simulink model "Diesel_UnitTest"  (Simulink 8.7)
settings: Solver=ode1  StartTime=0.0  StopTime=inf  FixedStep=Ts  MaxStep=1e-3  RelTol=1e-3
model workspace (MAT data in the model file):
  op_snapshot1 : opcond.OperatingPoint (value not decoded)
PostLoadFcn:
  | Test_init;
InitFcn:
  | Test_init;
values from neighbouring files (symbols this model uses):
  Ts = 100E-6    (= 0.0001)    [Test_init.m]
undefined symbols (not defined in the file or in its folder): Banshee_HWCtrl_IOs, Banshee_SEL751_Woodward_lib, fdesignblkfcn, gcbh, Left, type, V
libraries: simulink x11, rtio_opalrt_common x10, cables_lib x7, rtlab x6, breaker_lib x5, simulink_extras x3, Load_lib x3, PQFV_lib x2, powerlib x2, artemis x1, EasyGen3500_GensetSignalScaling_lib x1, HWController_Diesel_GenSet_4MVA_lib x1
(part 1 of 2)
settings Model: ARTEMISmethode_block_infos=$$__separator__$$Diesel_UnitTest/ARTEMIS Guide$$__separator__$$  Creator=RE25624  LastModifiedBy=g73labuser
settings SolverCC: ZeroCrossAlgorithm=Adaptive
settings DataIOCC: ExternalInput=getinputstruct(op_snapshot1)  InitialState=getstatestruct(op_snapshot1)  LimitDataPoints=off  MaxDataPoints=90060  SaveOutput=off  SignalLogging=off  DSMLogging=off  SaveTime=off  OutputSaveName=result
settings OptimizationCC: BlockReduction=off  OptimizeBlockIOStorage=off  BufferReuse=off  GlobalBufferReuse=off  ExpressionFolding=off  ExpressionDepthLimit=2147483647  LocalBlockOutputs=off
settings DebuggingCC: MaxConsecutiveZCsMsg=warning  IgnoredZcDiagnostic=none  MultiTaskRateTransMsg=warning  FcnCallInpInsideContextMsg=EnableAllAsWarning  ModelReferenceExtraNoncontSigs=warning  StateNameClashWarn=warning  StrictBusMsg=None
settings ModelReferenceCC: UpdateModelReferenceTargets=IfOutOfDate
settings SFSimCC: SFSimEcho=off
settings GRTTargetCC: CombineOutputUpdateFcns=off  GRTInterface=on

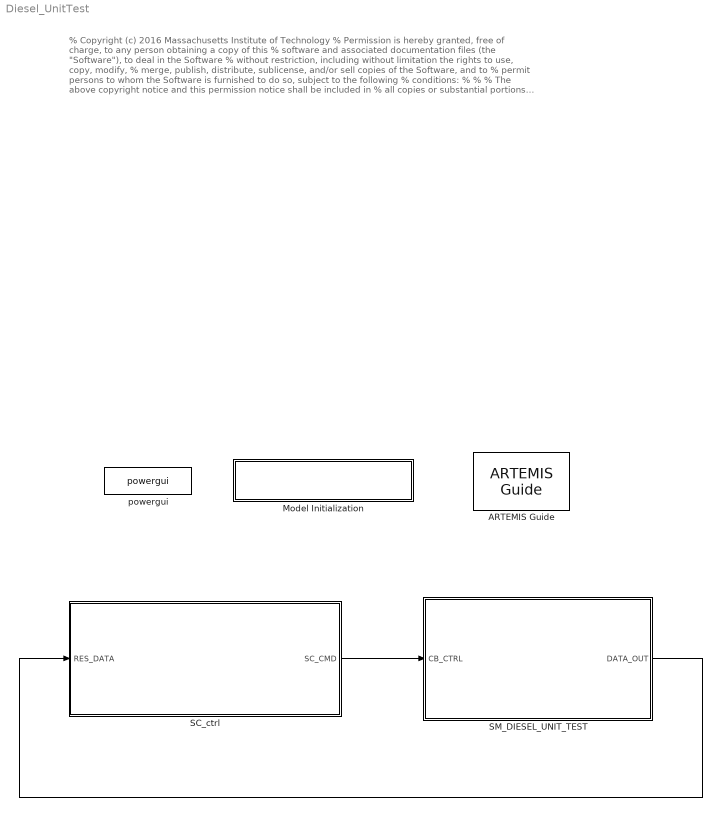
== system Diesel_UnitTest ==
  note: % Copyright (c) 2016 Massachusetts Institute of Technology
      | % Permission is hereby granted, free of charge, to any person obtaining a copy of this
      | % software and associated documentation files (the "Software"), to deal in the Software
      | % without restriction, including without limitation the rights to use, copy, modify,
      | % merge, publish, distribute, sublicense, and/or sell copies of the Software, and to
      | % permit persons to whom the Software is furnished to do so, subject to the following
      | % conditions:
      | %
      | %
      | % The above copyright notice and this permission notice shall be included in
      | % all copies or substantial portions of the Software.
      | %
      | % THE SOFTWARE IS PROVIDED "AS IS", WITHOUT WARRANTY OF ANY KIND, EXPRESS OR IMPLIED,
      | % INCLUDING BUT NOT LIMITED TO THE WARRANTIES OF MERCHANTABILITY, FITNESS FOR A
      | % PARTICULAR PURPOSE AND NONINFRINGEMENT. IN NO EVENT SHALL THE AUTHORS OR COPYRIGHT
      | % HOLDERS BE LIABLE FOR ANY CLAIM, DAMAGES OR OTHER LIABILITY, WHETHER IN AN ACTION
      | % OF CONTRACT, TORT OR OTHERWISE, ARISING FROM, OUT OF OR IN CONNECTION WITH THE
      | % SOFTWARE OR THE USE OR OTHER DEALINGS IN THE SOFTWARE.
      | %
      | %
      | %%
  ARTEMIS Guide : artemis/ARTEMIS/ARTEMIS Guide  Tag=FTSSmethode_opal_4hx0r99  Description=5.0_z1  lock=on  Ts=Ts  opt=art5  dyna=off  nb_perm=4  RT_fullcomp=off  ssn=on  ssn_itvc=off  ssn_ivic=off  ssn_ext=off  ssn_solver=Art5 with Backward Euler nodal interface  ssn_impulse=off  ssn_quasimpulse=off  ssn_impulse_loop=5  paraExtinctionThy=off  Thy_Impulse=on  dtc=Off  dtc_opt=normal  ao=on  simtype=off  ct_mac=off  lin_mov=off  lsp=[0.001 2]  spike_skip=Disabled  dtc_extra=1  dtc_sws=normal  dtc_pied=0.5  SPSRulesBlock=SPSRules  tre=on  ctmm=off  LF=off  dpl_type=ARTEMiS DPL  rlc_type=off  custom_type=off  para=on  ssn_ImpulseLoopBlockedStateUpdate=5  ssn_mov_iter_number=5  ssn_switch_iter_number=5  ssn_nib_type_verify=on  ssn_use_lu=on  ssn_use_ldlt=off
  Model Initialization : Subsystem  AncestorBlock=artemis/Tools /Misc/Model Initialization  mask(Model Functions){InitFcnX=Test_init;, prel=off, posl=on, inif=on, strf=off}
      mask prompts: InitFcnX "Initialisation"; prel "Preload Function"; posl "PostLoad Function"; inif "InitFcn"; strf "StartFcn"
      mask init:
      | currentBlock = gcb;
      | root = bdroot(currentBlock);
      | 
      | if ~strcmp(get_param(root,'BlockDiagramType'),'library')
      |     if prel==1
      |         set_param(root, 'PreLoadFcn', InitFcnX);
      |     else
      |         set_param(root, 'PreLoadFcn', '');
      |     end
      |     if inif==1
      |         set_param(root, 'InitFcn', InitFcnX);
      |     else
      |         set_param(root, 'InitFcn', '');
      |     end
      |     if strf==1
      |         set_param(root, 'StartFcn', InitFcnX);
      |     else
      |         set_param(root, 'StartFcn', '');
      |     end
      |     if posl==1
      |         set_param(root, 'PostLoadFcn', InitFcnX);
      |     else
      |         set_param(root, 'PostLoadFcn', '');
      |     end
      | end
      | 
      | pos = get_param(currentBlock, 'Position');
      | width = pos(3) - pos(1); height = pos(4) - pos(2);
      | txt = [ upper(root) '\n' '- InitFcn. . . . . '  get_param(root, 'InitFcn') ];
      settings: CopyFcn=set_param(gcb,'LinkStatus','inactive')
      mask Display: text(5, height*0.5, txt, 'horizontalAlignment', 'left', 'verticalAlignment', 'middle') ;
  SC_ctrl : Subsystem
  SM_DIESEL_UNIT_TEST : Subsystem
  powergui : powerlib/powergui  Priority=2  SimulationMode=Discrete  SolverType=Tustin  SampleTime=Ts  frequency=60  SPID=off  DisableSnubberDevices=off  DisableRonSwitches=off  DisableVfSwitches=off  SwTol=0  DisplayEquations=off  Interpol=off  ExternalGateDelay=off  methode=off  Ts=0  FunctionMessages=off  echomessages=off  HookPort=off  EnableUseOfTLC=off  x0status=blocks  frequencyindice=0  Pbase=100e6  ErrMax=1e-4  Iterations=50  UnitsV=kV  UnitsW=MW  buscounter=0  RestoreLinks=warning  ResistiveCurrentMeasurement=off  Frange=logspace(0,3,50)  Ylog=off  Xlog=off  ShowGrid=off  save=off  variable=ZData  structure=0  ZoomFFT=on  StartTime=0.0  cycles=2  DisplayStyle=off  fundamental=60  FreqAxis=off  MaxFrequency=1000  frequencyindicesteady=1  RmsSteady=1  display=off
  wires:
  SC_ctrl/1(SC_CMD) -> SM_DIESEL_UNIT_TEST/1(CB_CTRL)
  SM_DIESEL_UNIT_TEST/1(DATA_OUT) -> SC_ctrl/1(RES_DATA)

== system Diesel_UnitTest/Model Initialization ==

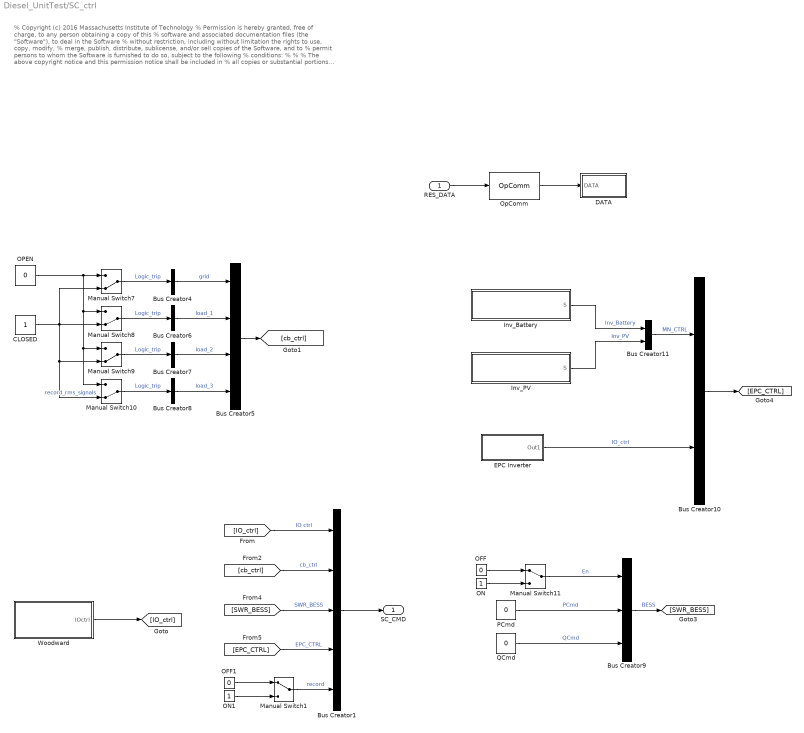
== system Diesel_UnitTest/SC_ctrl ==
  note: % Copyright (c) 2016 Massachusetts Institute of Technology
      | % Permission is hereby granted, free of charge, to any person obtaining a copy of this
      | % software and associated documentation files (the "Software"), to deal in the Software
      | % without restriction, including without limitation the rights to use, copy, modify,
      | % merge, publish, distribute, sublicense, and/or sell copies of the Software, and to
      | % permit persons to whom the Software is furnished to do so, subject to the following
      | % conditions:
      | %
      | %
      | % The above copyright notice and this permission notice shall be included in
      | % all copies or substantial portions of the Software.
      | %
      | % THE SOFTWARE IS PROVIDED "AS IS", WITHOUT WARRANTY OF ANY KIND, EXPRESS OR IMPLIED,
      | % INCLUDING BUT NOT LIMITED TO THE WARRANTIES OF MERCHANTABILITY, FITNESS FOR A
      | % PARTICULAR PURPOSE AND NONINFRINGEMENT. IN NO EVENT SHALL THE AUTHORS OR COPYRIGHT
      | % HOLDERS BE LIABLE FOR ANY CLAIM, DAMAGES OR OTHER LIABILITY, WHETHER IN AN ACTION
      | % OF CONTRACT, TORT OR OTHERWISE, ARISING FROM, OUT OF OR IN CONNECTION WITH THE
      | % SOFTWARE OR THE USE OR OTHER DEALINGS IN THE SOFTWARE.
      | %
      | %
      | %%
  RES_DATA : Inport
  Bus Creator1 : BusCreator  Inputs=5
  Bus Creator10 : BusCreator  Inputs=2
  Bus Creator11 : BusCreator  Inputs=2
  Bus Creator{4,6..8} (4 alike) : BusCreator  Inputs=1
  Bus Creator5 : BusCreator  Inputs=4
  Bus Creator9 : BusCreator  Inputs=3
  CLOSED : Constant
  DATA : Subsystem
  EPC Inverter : Subsystem
  Inv_Battery : Subsystem
  Inv_PV : Subsystem
  Manual Switch1 : ManualSwitch
  Manual Switch{7..10} (4 alike) : ManualSwitch  CurrentSetting=0
  Manual Switch11 : ManualSwitch
  OFF : Constant  Value=0
  OFF1 : Constant  Value=0
  ON : Constant
  ON1 : Constant
  OPEN : Constant  Value=0
  OpComm : rtlab/OpComm  nbport=1  groupe_acq=1  subsys_rate=0  st=0  Synchronization=on  Interpolation=on  Threshold=1.0  Missed_Data=off  Sim_Time=off  Samples=off  dynSigOut=off  from_console=0  warning_done=off  writeOpCommFile=off  Offset=off
  PCmd : Constant  Value=0  SampleTime=Ts
  QCmd : Constant  Value=0  SampleTime=Ts
  Woodward : Subsystem
  SC_CMD : Outport
  wires:
  Bus Creator1/1 -> SC_CMD/1
  [IO_ctrl] -> Bus Creator1/1  "IO ctrl"
  Woodward/1(IOctrl) -> [IO_ctrl]
  [cb_ctrl] -> Bus Creator1/2  "cb_ctrl"
  OpComm/1 -> DATA/1(DATA)
  RES_DATA/1 -> OpComm/1
  Manual Switch10/1 -> Bus Creator8/1  "Logic_trip"
  Manual Switch9/1 -> Bus Creator7/1  "Logic_trip"
  Bus Creator5/1 -> [cb_ctrl]
  Manual Switch8/1 -> Bus Creator6/1  "Logic_trip"
  Bus Creator4/1 -> Bus Creator5/1  "grid"
  Manual Switch7/1 -> Bus Creator4/1  "Logic_trip"
  Bus Creator8/1 -> Bus Creator5/4  "load_3"
  Bus Creator7/1 -> Bus Creator5/3  "load_2"
  Bus Creator6/1 -> Bus Creator5/2  "load_1"
  OPEN/1 -> Manual Switch7/1, Manual Switch8/1, Manual Switch9/1, Manual Switch10/1
  CLOSED/1 -> Manual Switch7/2, Manual Switch8/2, Manual Switch9/2, Manual Switch10/2  "record_rms_signals"
  Manual Switch11/1 -> Bus Creator9/1  "En"
  PCmd/1 -> Bus Creator9/2  "PCmd"
  QCmd/1 -> Bus Creator9/3  "QCmd"
  ON/1 -> Manual Switch11/2
  OFF/1 -> Manual Switch11/1
  Bus Creator9/1 -> [SWR_BESS]  "BESS"
  [SWR_BESS] -> Bus Creator1/3  "SWR_BESS"
  EPC Inverter/1(Out1) -> Bus Creator10/2  "IO_ctrl"
  Bus Creator10/1 -> [EPC_CTRL]
  [EPC_CTRL] -> Bus Creator1/4  "EPC_CTRL"
  Inv_Battery/1(S) -> Bus Creator11/1  "Inv_Battery"
  Bus Creator11/1 -> Bus Creator10/1  "MN_CTRL"
  Inv_PV/1(S) -> Bus Creator11/2  "Inv_PV"
  ON1/1 -> Manual Switch1/2
  OFF1/1 -> Manual Switch1/1
  Manual Switch1/1 -> Bus Creator1/5  "record"

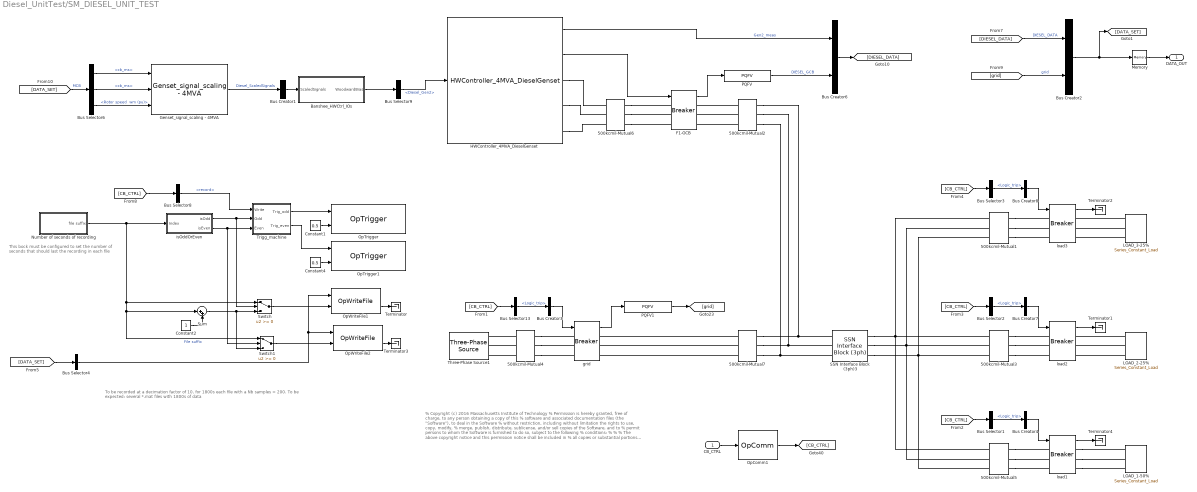
== system Diesel_UnitTest/SM_DIESEL_UNIT_TEST ==
  note: % Copyright (c) 2016 Massachusetts Institute of Technology
      | % Permission is hereby granted, free of charge, to any person obtaining a copy of this
      | % software and associated documentation files (the "Software"), to deal in the Software
      | % without restriction, including without limitation the rights to use, copy, modify,
      | % merge, publish, distribute, sublicense, and/or sell copies of the Software, and to
      | % permit persons to whom the Software is furnished to do so, subject to the following
      | % conditions:
      | %
      | %
      | % The above copyright notice and this permission notice shall be included in
      | % all copies or substantial portions of the Software.
      | %
      | % THE SOFTWARE IS PROVIDED "AS IS", WITHOUT WARRANTY OF ANY KIND, EXPRESS OR IMPLIED,
      | % INCLUDING BUT NOT LIMITED TO THE WARRANTIES OF MERCHANTABILITY, FITNESS FOR A
      | % PARTICULAR PURPOSE AND NONINFRINGEMENT. IN NO EVENT SHALL THE AUTHORS OR COPYRIGHT
      | % HOLDERS BE LIABLE FOR ANY CLAIM, DAMAGES OR OTHER LIABILITY, WHETHER IN AN ACTION
      | % OF CONTRACT, TORT OR OTHERWISE, ARISING FROM, OUT OF OR IN CONNECTION WITH THE
      | % SOFTWARE OR THE USE OR OTHER DEALINGS IN THE SOFTWARE.
      | %
      | %
      | %%
  note: This bock must be configured to set the number of
      | seconds that should last the recording in each file
  note: To be recorded at a decimation factor of 10,   for 1800s each file with a Nb samples = 200.
      | To be expected: several *.mat files with 1800s of data
  CB_CTRL : Inport
  500kcmil-Mutual1 : cables_lib/500kcmil-Mutual  length=500  par_sets=1  ratio=3
  500kcmil-Mutual{2,4,6..7} (4 alike) : cables_lib/500kcmil-Mutual  length=50  par_sets=1  ratio=3
  500kcmil-Mutual3 : cables_lib/500kcmil-Mutual  length=500  par_sets=1  ratio=3
  500kcmil-Mutual5 : cables_lib/500kcmil-Mutual  length=500  par_sets=1  ratio=3
  Banshee_HWCtrl_IOs : Subsystem  AncestorBlock=Banshee_SEL751_Woodward_lib/Banshee_HWCtrl_IOs
  Bus Creator{1,3..4,7..8} (5 alike) : BusCreator  Inputs=1
  Bus Creator2 : BusCreator  Inputs=2
  Bus Creator6 : BusCreator  Inputs=2
  Bus Selector1 : BusSelector  OutputSignals=cb_ctrl.load_1.Logic_trip
  Bus Selector13 : BusSelector  OutputSignals=cb_ctrl.grid.Logic_trip
  Bus Selector2 : BusSelector  OutputSignals=cb_ctrl.load_2.Logic_trip
  Bus Selector3 : BusSelector  OutputSignals=cb_ctrl.load_3.Logic_trip
  Bus Selector4 : BusSelector  OutputSignals="DIESEL_DATA.Gen2_meas.w.w.Rotor speed  wm (pu),DIESEL_DATA.Gen2_meas.Pm,DIESEL_DATA.DIESEL_GCB.VRMSLL,DIESEL_DATA.DIESEL_GCB.Freq,DIESEL_DATA.DIESEL_GCB.kw,DIESEL_DATA.DIESEL_GCB.kvar,DIESEL_DATA.DIESEL_GCB.cb_ms.Status,grid.VRMSLL,grid.Freq,grid.kw,grid.kvar,grid.cb_ms.Status"  OutputAsBus=on
  Bus Selector6 : BusSelector  OutputSignals="DIESEL_DATA.DIESEL_GCB.cb_ms,grid.cb_ms,DIESEL_DATA.Gen2_meas.w.w.Rotor speed  wm (pu)"
  Bus Selector8 : BusSelector  OutputSignals=record
  Bus Selector9 : BusSelector  OutputSignals=Diesel_Gen2
  Constant1 : Constant  Value=0.5
  Constant2 : Constant
  Constant4 : Constant  Value=0.5
  F1-GCB : breaker_lib/Breaker  Ts=Ts  mech_delay=cb_mech_delay
  Genset_signal_scaling - 4MVA : EasyGen3500_GensetSignalScaling_lib/Genset_signal_scaling - 4MVA  Vpk_mcb=11268  watt_mcb=3600000  Vpk_gcb=11268  watt_gcb=3600000  rated_rpm=1800  wm_noise_bias=0.02
  HWController_4MVA_DieselGenset : HWController_Diesel_GenSet_4MVA_lib/HWController_4MVA_DieselGenset
  LOAD_1-50% : Load_lib/Series_Constant_Load  v=13800  kVA=2000  pf=0.90
  LOAD_2-25% : Load_lib/Series_Constant_Load  v=13800  kVA=1000  pf=0.90
  LOAD_3-25% : Load_lib/Series_Constant_Load  v=13800  kVA=1000  pf=0.90
  Memory : Memory
  Number of seconds of recording : Subsystem  mask{time_s=1800}
      mask prompts: time_s "Time in seconds"
      mask help: Set the number of seconds that should last the recording in each file.
  OpComm1 : rtlab/OpComm  nbport=1  groupe_acq=1  subsys_rate=0  st=0  Synchronization=on  Interpolation=on  Threshold=1.0  Missed_Data=off  Sim_Time=off  Samples=off  dynSigOut=off  from_console=1  warning_done=off  writeOpCommFile=off  Offset=off
  OpTrigger : rtlab/DataLogging/OpTrigger  Trig_Type=TRIGGER SIGNAL >= TRIGGER LEVEL  Trig_Offset=0  Acq_Group=28
  OpTrigger1 : rtlab/DataLogging/OpTrigger  Trig_Type=TRIGGER SIGNAL >= TRIGGER LEVEL  Trig_Offset=0  Acq_Group=29
  OpWriteFile1 : rtlab/DataLogging/OpWriteFile  Static_File=off  varname=recVar  Filename=A_FILE_RECORDED_o.mat  rtpath='./'  nrtpath='.\'  Acq_Group=28  file_size=150000000  write_offline=off  Sim_Mode=off  Nb_Samples=1000  Buffer_size=0
      settings: Decimation=20
  OpWriteFile2 : rtlab/DataLogging/OpWriteFile  Static_File=off  varname=recVar  Filename=A_FILE_RECORDED_e.mat  rtpath='./'  nrtpath='.\'  Acq_Group=29  file_size=150000000  write_offline=off  Sim_Mode=off  Nb_Samples=1000  Buffer_size=0
      settings: Decimation=20
  PQFV : PQFV_lib/PQFV  VRMSLL=13800  Ts=Ts
  PQFV1 : PQFV_lib/PQFV  VRMSLL=13800  Ts=Ts
  SSN Interface Block (3ph)3 : ssn_lib/SSN Interface Block (3ph)  nb_phase=3  nb_port=2  p1_type=V-type(Left)  p2_type=V-type (Right)  p3_type=V-type(Left)  p4_type=V-type(Left)  p5_type=V-type(Left)  p6_type=V-type(Left)  p7_type=V-type(Left)  p8_type=V-type(Left)  p9_type=V-type(Left)  p10_type=V-type(Left)  p11_type=V-type(Left)  p12_type=V-type(Left)  p13_type=V-type(Left)  p14_type=V-type(Left)  p15_type=V-type(Left)  p16_type=V-type(Left)  I_port_shunt_resistance=1e9
  Sum : Sum  Inputs=|++
  Switch : Switch
  Switch1 : Switch
  Terminator{,1..4} (5 alike) : Terminator
  Three-Phase Source1 : powerlib/Electrical Sources/Three-Phase Source  InternalConnection=Yg  VoltagePhases=off  Voltage=13800 * 1.02  PhaseAngle=0  Voltage_phases=[25e3 25e3 25e3]/sqrt(3)  PhaseAngles_phases=[0 -120 +120]  Frequency=60  NonIdealSource=on  SpecifyImpedance=on  Resistance=0.8929  Inductance=16.58e-3  ShortCircuitLevel=2000e6  BaseVoltage=13800 * 1.02  XRratio=100  BusType=swing  Pref=0  Qref=0  Prefabc=[10e3, 10e3, 10e3]  Qrefabc=[0, 0, 0]  Qmin=-inf  Qmax=inf
  Trigg_machine : Subsystem
  grid : breaker_lib/Breaker  Ts=Ts  mech_delay=cb_mech_delay
  isOddOrEven : Subsystem
  load1 : breaker_lib/Breaker  Ts=Ts  mech_delay=cb_mech_delay
  load2 : breaker_lib/Breaker  Ts=Ts  mech_delay=cb_mech_delay
  load3 : breaker_lib/Breaker  Ts=Ts  mech_delay=cb_mech_delay
  DATA_OUT : Outport
  wires:
  Bus Selector9/1 -> HWController_4MVA_DieselGenset/1  "<Diesel_Gen2>"
  HWController_4MVA_DieselGenset/2 -> F1-GCB/1
  F1-GCB/1 -> PQFV/1
  Bus Creator6/1 -> [DIESEL_DATA]
  PQFV/1 -> Bus Creator6/2  "DIESEL_GCB"
  HWController_4MVA_DieselGenset/1 -> Bus Creator6/1  "Gen2_meas"
  Memory/1 -> DATA_OUT/1
  Bus Creator2/1 -> [DATA_SET], Memory/1
  [DIESEL_DATA] -> Bus Creator2/1  "DIESEL_DATA"
  [grid] -> Bus Creator2/2  "grid"
  [CB_CTRL] -> Bus Selector13/1
  Bus Selector13/1 -> Bus Creator3/1  "<Logic_trip>"
  Bus Creator3/1 -> grid/1
  grid/1 -> PQFV1/1
  PQFV1/1 -> [grid]
  [CB_CTRL] -> Bus Selector1/1
  Bus Selector1/1 -> Bus Creator4/1  "<Logic_trip>"
  Bus Creator4/1 -> load1/1
  [CB_CTRL] -> Bus Selector2/1
  Bus Selector2/1 -> Bus Creator7/1  "<Logic_trip>"
  Bus Creator7/1 -> load2/1
  [CB_CTRL] -> Bus Selector3/1
  Bus Selector3/1 -> Bus Creator8/1  "<Logic_trip>"
  Bus Creator8/1 -> load3/1
  load1/1 -> Terminator4/1
  load3/1 -> Terminator2/1
  load2/1 -> Terminator1/1
  Bus Selector4/1 -> OpWriteFile1/1, OpWriteFile2/1
  Trigg_machine/1(Trig_odd) -> OpTrigger/1
  Trigg_machine/2(Trig_even) -> OpTrigger1/1
  Constant1/1 -> OpTrigger/2
  Constant4/1 -> OpTrigger1/2
  isOddOrEven/1(isOdd) -> Switch/2, Trigg_machine/2(Odd)
  isOddOrEven/2(isEven) -> Switch1/2, Trigg_machine/3(Even)
  Switch/1 -> OpWriteFile1/2
  Switch1/1 -> OpWriteFile2/2
  Constant2/1 -> Sum/2
  Sum/1 -> Switch/3, Switch1/3
  Number of seconds of recording/1(file suffix) -> isOddOrEven/1(Index), Sum/1, Switch1/1, Switch/1  "File suffix"
  Bus Selector8/1 -> Trigg_machine/1(Write)  "<record>"
  OpWriteFile1/2 -> Terminator/1
  OpWriteFile2/2 -> Terminator3/1
  [CB_CTRL] -> Bus Selector8/1
  [DATA_SET] -> Bus Selector4/1
  CB_CTRL/1 -> OpComm1/1
  OpComm1/1 -> [CB_CTRL]
  [DATA_SET] -> Bus Selector6/1  "MCB"
  Bus Selector6/3 -> Genset_signal_scaling - 4MVA/3  "<Rotor speed  wm (pu)>"
  Bus Selector6/2 -> Genset_signal_scaling - 4MVA/2  "<cb_ms>"
  Bus Selector6/1 -> Genset_signal_scaling - 4MVA/1  "<cb_ms>"
  Genset_signal_scaling - 4MVA/1 -> Bus Creator1/1  "Diesel_ScaledSignals"
  Bus Creator1/1 -> Banshee_HWCtrl_IOs/1(ScaledSignals)
  Banshee_HWCtrl_IOs/1(WoodwardBias) -> Bus Selector9/1
  connections:
  500kcmil-Mutual6/RConn3 -- F1-GCB/LConn3
  500kcmil-Mutual6/RConn1 -- F1-GCB/LConn1
  500kcmil-Mutual6/RConn2 -- F1-GCB/LConn2
  HWController_4MVA_DieselGenset/RConn1 -- 500kcmil-Mutual6/LConn1
  HWController_4MVA_DieselGenset/RConn2 -- 500kcmil-Mutual6/LConn2
  HWController_4MVA_DieselGenset/RConn3 -- 500kcmil-Mutual6/LConn3
  500kcmil-Mutual4/LConn2 -- Three-Phase Source1/RConn2
  500kcmil-Mutual4/LConn1 -- Three-Phase Source1/RConn1
  500kcmil-Mutual4/LConn3 -- Three-Phase Source1/RConn3
  load1/RConn2 -- LOAD_1-50%/LConn2
  load1/RConn3 -- LOAD_1-50%/LConn3
  load1/RConn1 -- LOAD_1-50%/LConn1
  LOAD_2-25%/LConn1 -- load2/RConn1
  LOAD_2-25%/LConn2 -- load2/RConn2
  LOAD_2-25%/LConn3 -- load2/RConn3
  LOAD_3-25%/LConn3 -- load3/RConn3
  LOAD_3-25%/LConn1 -- load3/RConn1
  LOAD_3-25%/LConn2 -- load3/RConn2
  500kcmil-Mutual1/RConn3 -- load3/LConn3
  500kcmil-Mutual1/RConn2 -- load3/LConn2
  500kcmil-Mutual1/RConn1 -- load3/LConn1
  500kcmil-Mutual3/RConn1 -- load2/LConn1
  500kcmil-Mutual3/RConn3 -- load2/LConn3
  500kcmil-Mutual3/RConn2 -- load2/LConn2
  500kcmil-Mutual5/RConn1 -- load1/LConn1
  500kcmil-Mutual5/RConn3 -- load1/LConn3
  500kcmil-Mutual5/RConn2 -- load1/LConn2
  500kcmil-Mutual2/LConn3 -- F1-GCB/RConn3
  500kcmil-Mutual2/LConn2 -- F1-GCB/RConn2
  500kcmil-Mutual2/LConn1 -- F1-GCB/RConn1
  500kcmil-Mutual4/RConn2 -- grid/LConn2
  500kcmil-Mutual4/RConn3 -- grid/LConn3
  500kcmil-Mutual4/RConn1 -- grid/LConn1
  500kcmil-Mutual7/LConn2 -- grid/RConn2
  500kcmil-Mutual7/LConn3 -- grid/RConn3
  500kcmil-Mutual7/LConn1 -- grid/RConn1
  500kcmil-Mutual7/RConn3 -- 500kcmil-Mutual2/RConn3 -- SSN Interface Block (3ph)3/LConn3
  500kcmil-Mutual7/RConn2 -- 500kcmil-Mutual2/RConn2 -- SSN Interface Block (3ph)3/LConn2
  500kcmil-Mutual7/RConn1 -- 500kcmil-Mutual2/RConn1 -- SSN Interface Block (3ph)3/LConn1
  SSN Interface Block (3ph)3/RConn1 -- 500kcmil-Mutual1/LConn1 -- 500kcmil-Mutual5/LConn1 -- 500kcmil-Mutual3/LConn1
  SSN Interface Block (3ph)3/RConn3 -- 500kcmil-Mutual5/LConn3 -- 500kcmil-Mutual1/LConn3 -- 500kcmil-Mutual3/LConn3
  SSN Interface Block (3ph)3/RConn2 -- 500kcmil-Mutual5/LConn2 -- 500kcmil-Mutual1/LConn2 -- 500kcmil-Mutual3/LConn2

== system Diesel_UnitTest/SC_ctrl/DATA ==
  DATA : Inport
  Bus Selector : BusSelector  OutputSignals="DIESEL_DATA.DIESEL_GCB.Freq,DIESEL_DATA.Gen2_meas.w.w.Rotor speed  wm (pu),DIESEL_DATA.DIESEL_GCB.Vpu,DIESEL_DATA.DIESEL_GCB.kw,grid.kw,DIESEL_DATA.DIESEL_GCB.kvar,grid.kvar"
  Demux{,1..3} (4 alike) : Demux  Outputs=1
  Display : Display
  Mux : Mux  Inputs=2
  Mux1 : Mux  Inputs=2
  Mux2 : Mux  Inputs=2
  Scope : Scope  NumInputPorts=4
  wires:
  DATA/1 -> Bus Selector/1
  Bus Selector/1 -> Scope/1, Display/1  "<Freq>"
  Bus Selector/3 -> Mux/2  "<Vpu>"
  Bus Selector/2 -> Mux/1  "<Rotor speed  wm (pu)>"
  Mux/1 -> Scope/2
  Bus Selector/4 -> Demux/1  "<kw>"
  Bus Selector/5 -> Demux1/1  "<kw>"
  Mux1/1 -> Scope/3
  Bus Selector/6 -> Demux2/1  "<kvar>"
  Bus Selector/7 -> Demux3/1  "<kvar>"
  Mux2/1 -> Scope/4
  Demux/1 -> Mux1/1  "genset_kW"
  Demux1/1 -> Mux1/2  "grid_kW"
  Demux2/1 -> Mux2/1  "genset_kVAR"
  Demux3/1 -> Mux2/2  "grid_kW"

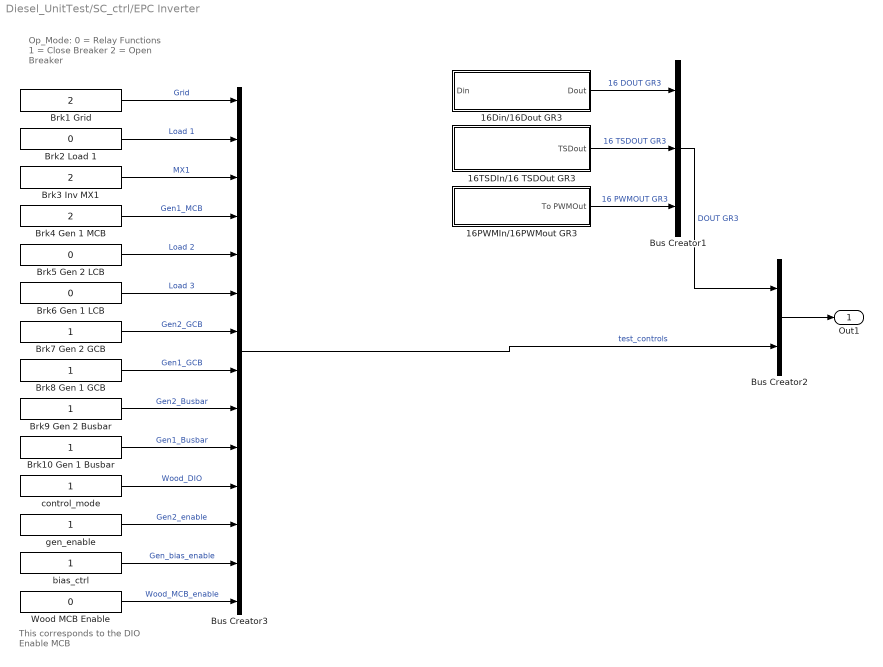
== system Diesel_UnitTest/SC_ctrl/EPC Inverter ==
  note: This corresponds to
      | the DIO Enable MCB
  note: Op_Mode:
      | 0 = Relay Functions
      | 1 = Close Breaker
      | 2 = Open Breaker
  16Din/16Dout GR3 : Subsystem
  16PWMIn/16PWMout GR3 : Subsystem
  16TSDIn/16 TSDOut GR3 : Subsystem
  Brk1 Grid : Constant  Value=2
  Brk10 Gen 1 Busbar : Constant
  Brk2 Load 1 : Constant  Value=0
  Brk3 Inv MX1 : Constant  Value=2
  Brk4 Gen 1 MCB : Constant  Value=2
  Brk5 Gen 2 LCB : Constant  Value=0
  Brk6 Gen 1 LCB : Constant  Value=0
  Brk7 Gen 2 GCB : Constant
  Brk8 Gen 1 GCB : Constant
  Brk9 Gen 2 Busbar : Constant
  Bus Creator1 : BusCreator  Inputs=3
  Bus Creator2 : BusCreator  Inputs=2
  Bus Creator3 : BusCreator  Inputs=14
  Wood MCB Enable : Constant  Value=0
  bias_ctrl : Constant
  control_mode : Constant
  gen_enable : Constant
  Out1 : Outport
  wires:
  Brk10 Gen 1 Busbar/1 -> Bus Creator3/10  "Gen1_Busbar"
  Brk9 Gen 2 Busbar/1 -> Bus Creator3/9  "Gen2_Busbar"
  Brk8 Gen 1 GCB/1 -> Bus Creator3/8  "Gen1_GCB"
  Brk7 Gen 2 GCB/1 -> Bus Creator3/7  "Gen2_GCB"
  Brk6 Gen 1 LCB/1 -> Bus Creator3/6  "Load 3"
  Brk5 Gen 2 LCB/1 -> Bus Creator3/5  "Load 2"
  Wood MCB Enable/1 -> Bus Creator3/14  "Wood_MCB_enable"
  Bus Creator2/1 -> Out1/1
  bias_ctrl/1 -> Bus Creator3/13  "Gen_bias_enable"
  gen_enable/1 -> Bus Creator3/12  "Gen2_enable"
  control_mode/1 -> Bus Creator3/11  "Wood_DIO"
  Brk4 Gen 1 MCB/1 -> Bus Creator3/4  "Gen1_MCB"
  Brk3 Inv MX1/1 -> Bus Creator3/3  "MX1"
  Brk2 Load 1/1 -> Bus Creator3/2  "Load 1"
  Brk1 Grid/1 -> Bus Creator3/1  "Grid"
  Bus Creator3/1 -> Bus Creator2/2  "test_controls"
  Bus Creator1/1 -> Bus Creator2/1  "DOUT GR3"
  16PWMIn/16PWMout GR3/1(To PWMOut) -> Bus Creator1/3  "16 PWMOUT GR3"
  16TSDIn/16 TSDOut GR3/1(TSDout) -> Bus Creator1/2  "16 TSDOUT GR3"
  16Din/16Dout GR3/1(Dout) -> Bus Creator1/1  "16 DOUT GR3"

== system Diesel_UnitTest/SC_ctrl/Inv_Battery ==
  note: Make this 1 to allow
      | the external signals.
  note: Remote Sense =>1
      | Use Remote Sense EPyQ
      | Sync or not => grid forming/grid following
  note: 0=> Local
      | 1=> Remote
  note: 0=> No Console
      | 1=> Console Ctrl
  note: 1 => Sig 1 is Bot then Sig 2 is Top
      | 0 => Sig 1 is Top then Sig 2 is Bot
  note: 0=> RTE
      | 1=> Simulink
  note: LSB
  note: MSB
  note: 1111: RTE TSD Signal Modulation External
      | 0111: RTE Signal Modulation Internal
      | X011: Sin Tri Modulatiion Internal
      | XX01: Digital Inputs
      | XXX0; Open Switches
  note: MCB
  note: GCB
  note: 1 => Closed
      | 0 => Open
  note: ~ 2.5 sec to get
      | to rated voltage
  note: RTE Internal
      | All 0 and one 1
  note: Internal = 0
      | External = 1
  Bus Creator : BusCreator  Inputs=8
  Bus Creator1 : BusCreator  Inputs=5
  Console : Constant  Value=0
  DC Contactor : Constant  Value=0
  Enable PWM{0..3} (4 alike) : Constant
  MX1 : Constant  Value=0
  MX2 : Constant  Value=0
  Precharge : Constant  Value=0
  Sense : Constant  Value=0
  Signal Mapping : Constant
  Simulink : Constant  Value=0
  S : Outport
  wires:
  Sense/1 -> Bus Creator/8  "LOCALvsREMOTE"
  Console/1 -> Bus Creator/7  "Console_Ctrl"
  Signal Mapping/1 -> Bus Creator1/5  "Ext_PWM_RTE_Signal"
  Simulink/1 -> Bus Creator/6  "RTEvsSPS"
  Enable PWM3/1 -> Bus Creator1/1
  Enable PWM2/1 -> Bus Creator1/2
  Enable PWM1/1 -> Bus Creator1/3
  Enable PWM0/1 -> Bus Creator1/4
  Bus Creator1/1 -> Bus Creator/1  "Enable PWM"
  MX2/1 -> Bus Creator/5  "MX2"
  MX1/1 -> Bus Creator/4  "MX1"
  DC Contactor/1 -> Bus Creator/3  "DC_Contactor"
  Precharge/1 -> Bus Creator/2  "Precharge"
  Bus Creator/1 -> S/1

== system Diesel_UnitTest/SC_ctrl/Inv_PV ==
  note: Make this 1 to allow
      | the external signals.
  note: Remote Sense =>1
      | Use Remote Sense EPyQ
      | Sync or not => grid forming/grid following
  note: 0=> Local
      | 1=> Remote
  note: 0=> No Console
      | 1=> Console Ctrl
  note: 1 => Sig 1 is Bot then Sig 2 is Top
      | 0 => Sig 1 is Top then Sig 2 is Bot
  note: 0=> RTE
      | 1=> Simulink
  note: LSB
  note: MSB
  note: 1111: RTE TSD Signal Modulation External
      | 0111: RTE Signal Modulation Internal
      | X011: Sin Tri Modulatiion Internal
      | XX01: Digital Inputs
      | XXX0; Open Switches
  note: MCB
  note: GCB
  note: 1 => Closed
      | 0 => Open
  note: ~ 2.5 sec to get
      | to rated voltage
  note: RTE Internal
      | All 0 and one 1
  note: Internal = 0
      | External = 1
  Bus Creator : BusCreator  Inputs=8
  Bus Creator1 : BusCreator  Inputs=5
  Console : Constant  Value=0
  DC Contactor : Constant  Value=0
  Enable PWM{0..3} (4 alike) : Constant
  MX1 : Constant  Value=0
  MX2 : Constant  Value=0
  Precharge : Constant  Value=0
  Sense : Constant  Value=0
  Signal Mapping : Constant
  Simulink : Constant  Value=0
  S : Outport
  wires:
  Sense/1 -> Bus Creator/8  "LOCALvsREMOTE"
  Console/1 -> Bus Creator/7  "Console_Ctrl"
  Signal Mapping/1 -> Bus Creator1/5  "Ext_PWM_RTE_Signal"
  Simulink/1 -> Bus Creator/6  "RTEvsSPS"
  Enable PWM3/1 -> Bus Creator1/1
  Enable PWM2/1 -> Bus Creator1/2
  Enable PWM1/1 -> Bus Creator1/3
  Enable PWM0/1 -> Bus Creator1/4
  Bus Creator1/1 -> Bus Creator/1  "Enable PWM"
  MX2/1 -> Bus Creator/5  "MX2"
  MX1/1 -> Bus Creator/4  "MX1"
  DC Contactor/1 -> Bus Creator/3  "DC_Contactor"
  Precharge/1 -> Bus Creator/2  "Precharge"
  Bus Creator/1 -> S/1

== system Diesel_UnitTest/SC_ctrl/Woodward ==
  16Din/16Dout GR3 : Subsystem
  Bus Creator2 : BusCreator  Inputs=1
  IOctrl : Outport
  wires:
  16Din/16Dout GR3/1(Dout) -> Bus Creator2/1  "16 DOUT GR3"
  Bus Creator2/1 -> IOctrl/1  "IO ctrl"

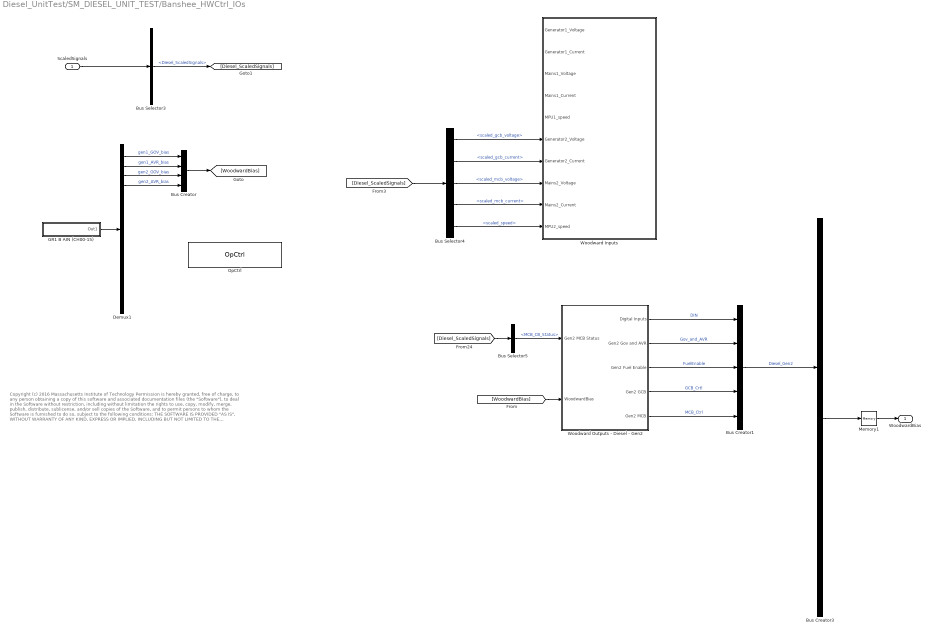
== system Diesel_UnitTest/SM_DIESEL_UNIT_TEST/Banshee_HWCtrl_IOs ==
  note: Copyright (c) 2016 Massachusetts Institute of Technology
      | Permission is hereby granted, free of charge, to any person obtaining a copy of this software and associated documentation files (the "Software"), to deal
      | in the Software without restriction, including without limitation the rights to use, copy, modify, merge, publish, distribute, sublicense, and/or sell copies of the
      | Software, and to permit persons to whom the Software is furnished to do so, subject to the following conditions:
      |
      | THE SOFTWARE IS PROVIDED "AS IS", WITHOUT WARRANTY OF ANY KIND, EXPRESS OR IMPLIED, INCLUDING BUT NOT LIMITED TO THE
      | WARRANTIES OF MERCHANTABILITY, FITNESS FOR A PARTICULAR PURPOSE AND NONINFRINGEMENT. IN NO EVENT SHALL THE AUTHORS
      | OR COPYRIGHT HOLDERS BE LIABLE FOR ANY CLAIM, DAMAGES OR OTHER LIABILITY, WHETHER IN AN ACTION OF CONTRACT, TORT OR
      | OTHERWISE, ARISING FROM, OUT OF OR IN CONNECTION WITH THE SOFTWARE OR THE USE OR OTHER DEALINGS IN THE SOFTWARE
  ScaledSignals : Inport
  Bus Creator : BusCreator  Inputs=4
  Bus Creator1 : BusCreator  Inputs=5
  Bus Creator3 : BusCreator  Inputs=4
  Bus Selector3 : BusSelector  OutputSignals=Diesel_ScaledSignals
  Bus Selector4 : BusSelector  OutputSignals=scaled_gcb_voltage,scaled_gcb_current,scaled_mcb_voltage,scaled_mcb_current,scaled_speed
  Bus Selector5 : BusSelector  OutputSignals=MCB_CB_Status
  Demux1 : Demux  Outputs=16
  GR1 B AIN (CH00-15) : Subsystem
  Memory1 : Memory
  OpCtrl : rtio_opalrt_common/OpCtrl  CtrlName='OpCtrl'  boardid=0  BitstreamFilename=VC707_2-EX-0001-2_3_2_20-48AIO16DIO16DIOSel-02-01.bin  numconfig=-1  mode=Master  externalClock=off  decimRtsi=0  calibIO=off  SampleTime=0  loadinport=-1  BoardType=VC707  SecondaryPresent=off  sync_type=Audio
  Woodward Inputs : Subsystem
  Woodward Outputs - Diesel - Gen2 : Subsystem
  WoodwardBias : Outport
  wires:
  Bus Creator/1 -> [WoodwardBias]
  Memory1/1 -> WoodwardBias/1
  Woodward Outputs - Diesel - Gen2/1(Digital Inputs) -> Bus Creator1/1  "DIN"
  Bus Creator3/1 -> Memory1/1
  Bus Creator1/1 -> Bus Creator3/2  "Diesel_Gen2"
  Woodward Outputs - Diesel - Gen2/5(Gen2 MCB) -> Bus Creator1/5  "MCB_Ctrl"
  Woodward Outputs - Diesel - Gen2/4(Gen2 GCB) -> Bus Creator1/4  "GCB_Crtl"
  Woodward Outputs - Diesel - Gen2/3(Gen2 Fuel Enable) -> Bus Creator1/3  "FuelEnable"
  Woodward Outputs - Diesel - Gen2/2(Gen2 Gov and AVR) -> Bus Creator1/2  "Gov_and_AVR"
  [Diesel_ScaledSignals] -> Bus Selector5/1
  [WoodwardBias] -> Woodward Outputs - Diesel - Gen2/2(WoodwardBias)
  Bus Selector5/1 -> Woodward Outputs - Diesel - Gen2/1(Gen2 MCB Status)  "<MCB_CB_Status>"
  Demux1/4 -> Bus Creator/4  "gen2_AVR_bias"
  Demux1/3 -> Bus Creator/3  "gen2_GOV_bias"
  Demux1/2 -> Bus Creator/2  "gen1_AVR_bias"
  Demux1/1 -> Bus Creator/1  "gen1_GOV_bias"
  GR1 B AIN (CH00-15)/1(Out1) -> Demux1/1
  Bus Selector4/5 -> Woodward Inputs/10(MPU2_speed)  "<scaled_speed>"
  Bus Selector4/4 -> Woodward Inputs/9(Mains2_Current)  "<scaled_mcb_current>"
  Bus Selector4/3 -> Woodward Inputs/8(Mains2_Voltage)  "<scaled_mcb_voltage>"
  Bus Selector4/2 -> Woodward Inputs/7(Generator2_Current)  "<scaled_gcb_current>"
  Bus Selector4/1 -> Woodward Inputs/6(Generator2_Voltage)  "<scaled_gcb_voltage>"
  [Diesel_ScaledSignals] -> Bus Selector4/1
  Bus Selector3/1 -> [Diesel_ScaledSignals]  "<Diesel_ScaledSignals>"
  ScaledSignals/1 -> Bus Selector3/1

== system Diesel_UnitTest/SM_DIESEL_UNIT_TEST/Number of seconds of recording ==
  Compare To Constant1 : simulink/Logic and Bit Operations/Compare To Constant  relop=>=  const=time_s  OutDataTypeStr=boolean
  Increment : Subsystem
  Integrator : Integrator  ExternalReset=rising
  Memory : Memory
  Slope : Constant
  file suffix : Outport
  wires:
  Slope/1 -> Integrator/1
  Integrator/1 -> Compare To Constant1/1
  Compare To Constant1/1 -> Memory/1, Increment/Trigger  "limit reached"
  Memory/1 -> Integrator/2
  Increment/1(Out1) -> file suffix/1

== system Diesel_UnitTest/SM_DIESEL_UNIT_TEST/Trigg_machine ==
  Write : Inport
  Odd : Inport  Port=2
  Even : Inport  Port=3
  Bitwise Operator : simulink/Logic and Bit Operations/Bitwise Operator  logicop=AND  UseBitMask=off  NumInputPorts=2  BitMask=bin2dec('11011001')  BitMaskRealWorld=Stored Integer
  Bitwise Operator1 : simulink/Logic and Bit Operations/Bitwise Operator  logicop=AND  UseBitMask=off  NumInputPorts=2  BitMask=bin2dec('11011001')  BitMaskRealWorld=Stored Integer
  Data Type Conversion : DataTypeConversion
  Data Type Conversion1 : DataTypeConversion
  Double2uint8 : DataTypeConversion
  Trig_odd : Outport
  Trig_even : Outport  Port=2
  wires:
  Double2uint8/1 -> Bitwise Operator1/1, Bitwise Operator/2
  Write/1 -> Double2uint8/1
  Odd/1 -> Bitwise Operator/1
  Data Type Conversion1/1 -> Trig_even/1
  Data Type Conversion/1 -> Trig_odd/1
  Even/1 -> Bitwise Operator1/2
  Bitwise Operator1/1 -> Data Type Conversion1/1
  Bitwise Operator/1 -> Data Type Conversion/1

== system Diesel_UnitTest/SM_DIESEL_UNIT_TEST/isOddOrEven ==
  note: Si cette différence est égale à 0, c'est que le
      | nombre en entrée est pair, sinon c'est qu'il est impair.
  note: Effectuer la différence entre le nombre en entrée,
      | et sa moitié arrondie multipliée par 2.
  Index : Inport
  Compare To Zero : simulink/Logic and Bit Operations/Compare To Zero  relop=~=  OutDataTypeStr=boolean  ZeroCross=off
  Compare To Zero1 : simulink/Logic and Bit Operations/Compare To Zero  relop===  OutDataTypeStr=boolean  ZeroCross=off
  Constant3 : Constant  Value=2
  Divide : Product  Inputs=*/  OutDataTypeStr=double
  Produit : Product  Inputs=**  OutDataTypeStr=double
  Rounding Function : Rounding
  Sum : Sum  Inputs=|+-
  isOdd : Outport
  isEven : Outport  Port=2
  wires:
  Compare To Zero1/1 -> isEven/1
  Compare To Zero/1 -> isOdd/1
  Sum/1 -> Compare To Zero1/1, Compare To Zero/1
  Produit/1 -> Sum/2
  Rounding Function/1 -> Produit/1
  Index/1 -> Sum/1, Divide/1
  Divide/1 -> Rounding Function/1
  Constant3/1 -> Produit/2, Divide/2

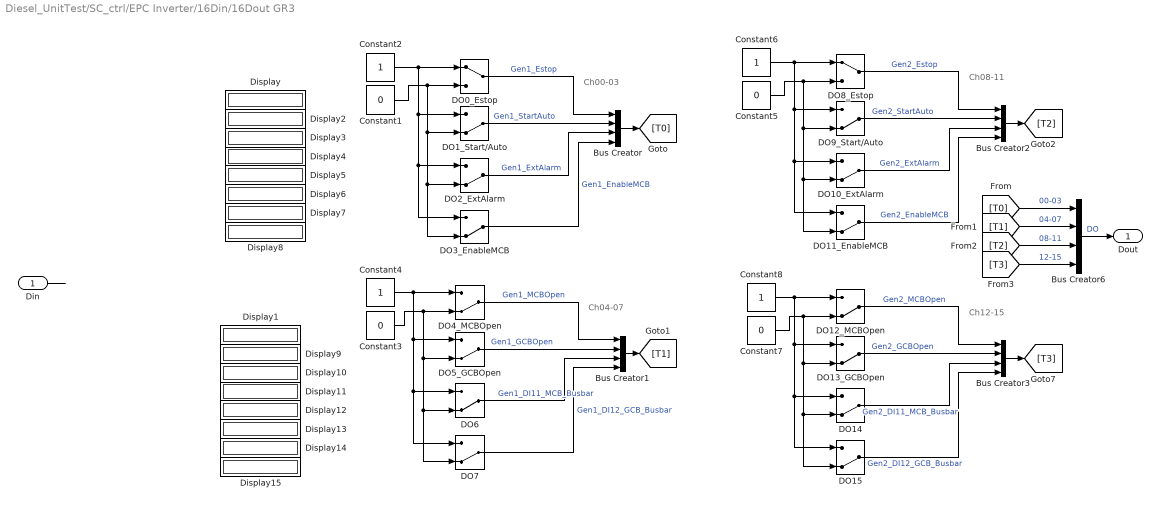
== system Diesel_UnitTest/SC_ctrl/EPC Inverter/16Din/16Dout GR3 ==
  note: Ch12-15
  note: Ch08-11
  note: Ch04-07
  note: Ch00-03
  Din : Inport
  Bus Creator{,1..3,6} (5 alike) : BusCreator  Inputs=4
  Constant{1,3,5,7} (4 alike) : Constant  Value=0
  Constant{2,4,6,8} (4 alike) : Constant
  DO0_Estop : ManualSwitch
  DO10_ExtAlarm : ManualSwitch  CurrentSetting=0
  DO11_EnableMCB : ManualSwitch  CurrentSetting=0
  DO12_MCBOpen : ManualSwitch  CurrentSetting=0
  DO13_GCBOpen : ManualSwitch  CurrentSetting=0
  DO{6..7,14..15} (4 alike) : ManualSwitch  CurrentSetting=0
  DO1_Start/Auto : ManualSwitch  CurrentSetting=0
  DO2_ExtAlarm : ManualSwitch  CurrentSetting=0
  DO3_EnableMCB : ManualSwitch  CurrentSetting=0
  DO4_MCBOpen : ManualSwitch  CurrentSetting=0
  DO5_GCBOpen : ManualSwitch  CurrentSetting=0
  DO8_Estop : ManualSwitch
  DO9_Start/Auto : ManualSwitch  CurrentSetting=0
  Display{,1..15} (16 alike) : Display
  Dout : Outport
  wires:
  ? -> Display7/1  "<Gen1_Alarm_AB>"
  ? -> Display4/1  "<Gen1_Open_GCB>"
  ? -> Display15/1  "<Gen2_Alarm_CF>"
  ? -> Display14/1  "<Gen2_Alarm_AB>"
  ? -> Display13/1  "<Gen2_Open_MCB>"
  ? -> Display12/1  "<Gen2_Close_MCB>"
  ? -> Display11/1  "<Gen2_Open_GCB>"
  ? -> Display10/1  "<Gen2_Close_GCB>"
  ? -> Display9/1  "<Gen2_Fuel>"
  ? -> Display1/1  "<Gen2_Starter>"
  ? -> ?  "<DI_CH08-15>"
  ? -> Display8/1  "<Gen1_Alarm_CF>"
  ? -> Display6/1  "<Gen1_Open_MCB>"
  ? -> Display5/1  "<Gen1_Close_MCB>"
  ? -> Display3/1  "<Gen1_Close_GCB>"
  ? -> Display2/1  "<Gen1_Fuel>"
  ? -> Display/1  "<Gen1_Starter>"
  ? -> ?  "<DI_CH00-07>"
  Din/1 -> ?
  [T3] -> Bus Creator6/4  "12-15"
  [T2] -> Bus Creator6/3  "08-11"
  [T1] -> Bus Creator6/2  "04-07"
  [T0] -> Bus Creator6/1  "00-03"
  Bus Creator2/1 -> [T2]
  Bus Creator3/1 -> [T3]
  Bus Creator1/1 -> [T1]
  Bus Creator/1 -> [T0]
  DO15/1 -> Bus Creator3/4  "Gen2_DI12_GCB_Busbar"
  DO14/1 -> Bus Creator3/3  "Gen2_DI11_MCB_Busbar"
  DO13_GCBOpen/1 -> Bus Creator3/2  "Gen2_GCBOpen"
  DO12_MCBOpen/1 -> Bus Creator3/1  "Gen2_MCBOpen"
  Constant7/1 -> DO12_MCBOpen/2, DO13_GCBOpen/2, DO15/2, DO14/2
  Constant8/1 -> DO12_MCBOpen/1, DO13_GCBOpen/1, DO15/1, DO14/1
  DO11_EnableMCB/1 -> Bus Creator2/4  "Gen2_EnableMCB"
  DO10_ExtAlarm/1 -> Bus Creator2/3  "Gen2_ExtAlarm"
  DO9_Start/Auto/1 -> Bus Creator2/2  "Gen2_StartAuto"
  DO8_Estop/1 -> Bus Creator2/1  "Gen2_Estop"
  Constant5/1 -> DO10_ExtAlarm/2, DO11_EnableMCB/2, DO9_Start/Auto/2, DO8_Estop/2
  Constant6/1 -> DO10_ExtAlarm/1, DO11_EnableMCB/1, DO9_Start/Auto/1, DO8_Estop/1
  DO7/1 -> Bus Creator1/4  "Gen1_DI12_GCB_Busbar"
  DO6/1 -> Bus Creator1/3  "Gen1_DI11_MCB_Busbar"
  DO5_GCBOpen/1 -> Bus Creator1/2  "Gen1_GCBOpen"
  DO4_MCBOpen/1 -> Bus Creator1/1  "Gen1_MCBOpen"
  Constant3/1 -> DO4_MCBOpen/2, DO5_GCBOpen/2, DO7/2, DO6/2
  Constant4/1 -> DO4_MCBOpen/1, DO5_GCBOpen/1, DO7/1, DO6/1
  DO3_EnableMCB/1 -> Bus Creator/4  "Gen1_EnableMCB"
  DO2_ExtAlarm/1 -> Bus Creator/3  "Gen1_ExtAlarm"
  DO1_Start/Auto/1 -> Bus Creator/2  "Gen1_StartAuto"
  DO0_Estop/1 -> Bus Creator/1  "Gen1_Estop"
  Constant1/1 -> DO2_ExtAlarm/2, DO3_EnableMCB/2, DO1_Start/Auto/2, DO0_Estop/2
  Constant2/1 -> DO2_ExtAlarm/1, DO3_EnableMCB/1, DO1_Start/Auto/1, DO0_Estop/1
  Bus Creator6/1 -> Dout/1  "DO"

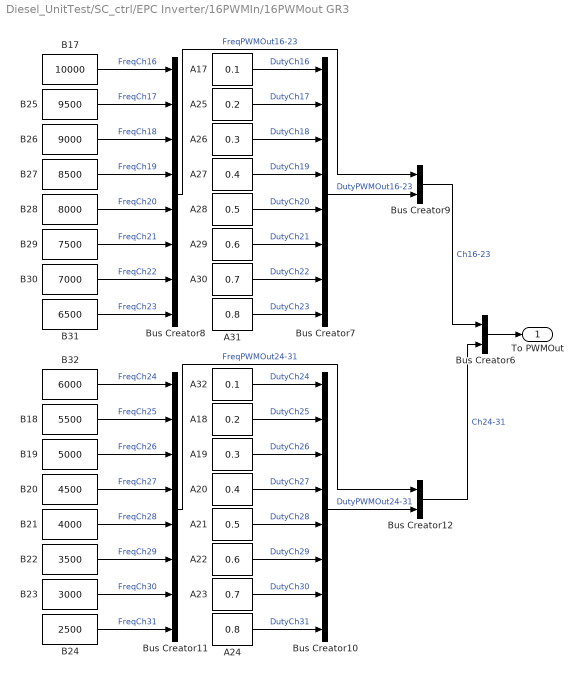
== system Diesel_UnitTest/SC_ctrl/EPC Inverter/16PWMIn/16PWMout GR3 ==
  A17 : Constant  Value=0.1
  A18 : Constant  Value=0.2
  A19 : Constant  Value=0.3
  A20 : Constant  Value=0.4
  A21 : Constant  Value=0.5
  A22 : Constant  Value=0.6
  A23 : Constant  Value=0.7
  A24 : Constant  Value=0.8
  A25 : Constant  Value=0.2
  A26 : Constant  Value=0.3
  A27 : Constant  Value=0.4
  A28 : Constant  Value=0.5
  A29 : Constant  Value=0.6
  A30 : Constant  Value=0.7
  A31 : Constant  Value=0.8
  A32 : Constant  Value=0.1
  B17 : Constant  Value=10000
  B18 : Constant  Value=5500
  B19 : Constant  Value=5000
  B20 : Constant  Value=4500
  B21 : Constant  Value=4000
  B22 : Constant  Value=3500
  B23 : Constant  Value=3000
  B24 : Constant  Value=2500
  B25 : Constant  Value=9500
  B26 : Constant  Value=9000
  B27 : Constant  Value=8500
  B28 : Constant  Value=8000
  B29 : Constant  Value=7500
  B30 : Constant  Value=7000
  B31 : Constant  Value=6500
  B32 : Constant  Value=6000
  Bus Creator{7..8,10..11} (4 alike) : BusCreator  Inputs=8
  Bus Creator12 : BusCreator  Inputs=2
  Bus Creator6 : BusCreator  Inputs=2
  Bus Creator9 : BusCreator  Inputs=2
  To PWMOut : Outport
  wires:
  Bus Creator9/1 -> Bus Creator6/1  "Ch16-23"
  Bus Creator12/1 -> Bus Creator6/2  "Ch24-31"
  Bus Creator11/1 -> Bus Creator12/1  "FreqPWMOut24-31"
  Bus Creator10/1 -> Bus Creator12/2  "DutyPWMOut24-31"
  B24/1 -> Bus Creator11/8  "FreqCh31"
  B23/1 -> Bus Creator11/7  "FreqCh30"
  B22/1 -> Bus Creator11/6  "FreqCh29"
  B21/1 -> Bus Creator11/5  "FreqCh28"
  B20/1 -> Bus Creator11/4  "FreqCh27"
  B19/1 -> Bus Creator11/3  "FreqCh26"
  B18/1 -> Bus Creator11/2  "FreqCh25"
  B32/1 -> Bus Creator11/1  "FreqCh24"
  A24/1 -> Bus Creator10/8  "DutyCh31"
  A23/1 -> Bus Creator10/7  "DutyCh30"
  A22/1 -> Bus Creator10/6  "DutyCh29"
  A21/1 -> Bus Creator10/5  "DutyCh28"
  A20/1 -> Bus Creator10/4  "DutyCh27"
  A19/1 -> Bus Creator10/3  "DutyCh26"
  A18/1 -> Bus Creator10/2  "DutyCh25"
  A32/1 -> Bus Creator10/1  "DutyCh24"
  Bus Creator8/1 -> Bus Creator9/1  "FreqPWMOut16-23"
  Bus Creator7/1 -> Bus Creator9/2  "DutyPWMOut16-23"
  B31/1 -> Bus Creator8/8  "FreqCh23"
  B30/1 -> Bus Creator8/7  "FreqCh22"
  B29/1 -> Bus Creator8/6  "FreqCh21"
  B28/1 -> Bus Creator8/5  "FreqCh20"
  B27/1 -> Bus Creator8/4  "FreqCh19"
  B26/1 -> Bus Creator8/3  "FreqCh18"
  B25/1 -> Bus Creator8/2  "FreqCh17"
  B17/1 -> Bus Creator8/1  "FreqCh16"
  A31/1 -> Bus Creator7/8  "DutyCh23"
  A30/1 -> Bus Creator7/7  "DutyCh22"
  A29/1 -> Bus Creator7/6  "DutyCh21"
  A28/1 -> Bus Creator7/5  "DutyCh20"
  A27/1 -> Bus Creator7/4  "DutyCh19"
  A26/1 -> Bus Creator7/3  "DutyCh18"
  A25/1 -> Bus Creator7/2  "DutyCh17"
  A17/1 -> Bus Creator7/1  "DutyCh16"
  Bus Creator6/1 -> To PWMOut/1

== system Diesel_UnitTest/SC_ctrl/EPC Inverter/16TSDIn/16 TSDOut GR3 ==
  Bus Creator1 : BusCreator  Inputs=3
  Din/Dout ch16-23 : Subsystem
  Din/Dout ch24-31 : Subsystem
  Dout state ctrl : Subsystem
  TSDout : Outport
  wires:
  Bus Creator1/1 -> TSDout/1
  Dout state ctrl/1(Event State OUT) -> Bus Creator1/3  "states"
  Din/Dout ch16-23/1(Out1) -> Bus Creator1/1  "times CH16-23"
  Din/Dout ch24-31/1(Out1) -> Bus Creator1/2  "times CH24-31"

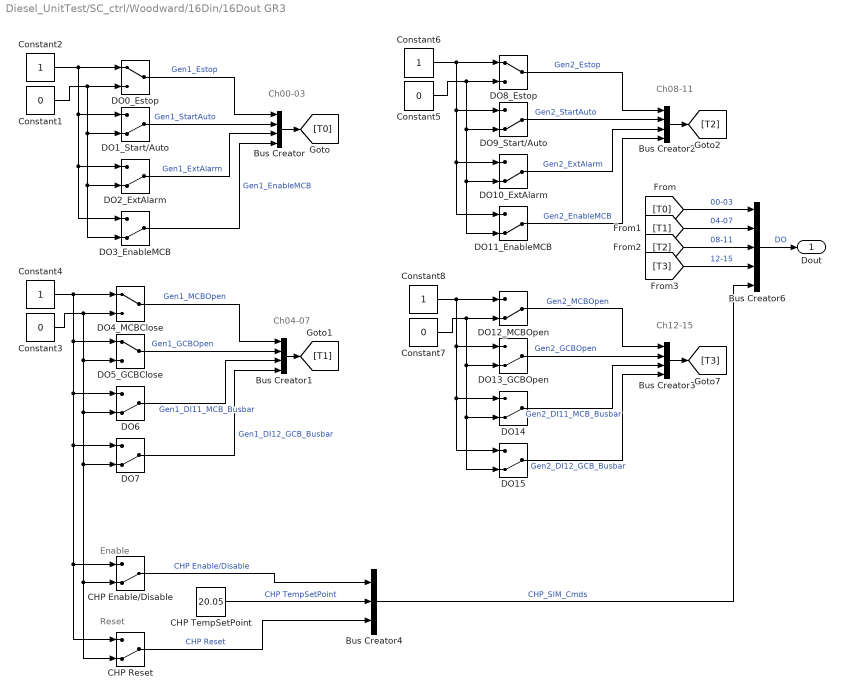
== system Diesel_UnitTest/SC_ctrl/Woodward/16Din/16Dout GR3 ==
  note: Ch00-03
  note: Ch04-07
  note: Ch08-11
  note: Ch12-15
  note: Enable
  note: Reset
  Bus Creator{,1..3} (4 alike) : BusCreator  Inputs=4
  Bus Creator4 : BusCreator  Inputs=3
  Bus Creator6 : BusCreator  Inputs=5
  CHP Enable/Disable : ManualSwitch  CurrentSetting=0
  CHP Reset : ManualSwitch  CurrentSetting=0
  CHP TempSetPoint : Constant  Value=20.05
  Constant{1,3,5,7} (4 alike) : Constant  Value=0
  Constant{2,4,6,8} (4 alike) : Constant
  DO0_Estop : ManualSwitch
  DO10_ExtAlarm : ManualSwitch  CurrentSetting=0
  DO11_EnableMCB : ManualSwitch  CurrentSetting=0
  DO12_MCBOpen : ManualSwitch  CurrentSetting=0
  DO13_GCBOpen : ManualSwitch  CurrentSetting=0
  DO{6..7,14..15} (4 alike) : ManualSwitch  CurrentSetting=0
  DO1_Start/Auto : ManualSwitch  CurrentSetting=0
  DO2_ExtAlarm : ManualSwitch  CurrentSetting=0
  DO3_EnableMCB : ManualSwitch  CurrentSetting=0
  DO4_MCBClose : ManualSwitch
  DO5_GCBClose : ManualSwitch
  DO8_Estop : ManualSwitch
  DO9_Start/Auto : ManualSwitch  CurrentSetting=0
  Dout : Outport
  wires:
  Bus Creator4/1 -> Bus Creator6/5  "CHP_SIM_Cmds"
  CHP Reset/1 -> Bus Creator4/3  "CHP Reset"
  CHP TempSetPoint/1 -> Bus Creator4/2  "CHP TempSetPoint"
  CHP Enable/Disable/1 -> Bus Creator4/1  "CHP Enable/Disable"
  Bus Creator6/1 -> Dout/1  "DO"
  Constant2/1 -> DO0_Estop/1, DO1_Start/Auto/1, DO3_EnableMCB/1, DO2_ExtAlarm/1
  Constant1/1 -> DO0_Estop/2, DO1_Start/Auto/2, DO3_EnableMCB/2, DO2_ExtAlarm/2
  DO0_Estop/1 -> Bus Creator/1  "Gen1_Estop"
  DO1_Start/Auto/1 -> Bus Creator/2  "Gen1_StartAuto"
  DO2_ExtAlarm/1 -> Bus Creator/3  "Gen1_ExtAlarm"
  DO3_EnableMCB/1 -> Bus Creator/4  "Gen1_EnableMCB"
  Constant4/1 -> DO6/1, DO7/1, CHP Enable/Disable/1, CHP Reset/1, DO5_GCBClose/1, DO4_MCBClose/1
  Constant3/1 -> DO6/2, CHP Enable/Disable/2, CHP Reset/2, DO7/2, DO5_GCBClose/2, DO4_MCBClose/2
  DO4_MCBClose/1 -> Bus Creator1/1  "Gen1_MCBOpen"
  DO5_GCBClose/1 -> Bus Creator1/2  "Gen1_GCBOpen"
  DO6/1 -> Bus Creator1/3  "Gen1_DI11_MCB_Busbar"
  DO7/1 -> Bus Creator1/4  "Gen1_DI12_GCB_Busbar"
  Constant6/1 -> DO8_Estop/1, DO9_Start/Auto/1, DO11_EnableMCB/1, DO10_ExtAlarm/1
  Constant5/1 -> DO8_Estop/2, DO9_Start/Auto/2, DO11_EnableMCB/2, DO10_ExtAlarm/2
  DO8_Estop/1 -> Bus Creator2/1  "Gen2_Estop"
  DO9_Start/Auto/1 -> Bus Creator2/2  "Gen2_StartAuto"
  DO10_ExtAlarm/1 -> Bus Creator2/3  "Gen2_ExtAlarm"
  DO11_EnableMCB/1 -> Bus Creator2/4  "Gen2_EnableMCB"
  Constant8/1 -> DO14/1, DO15/1, DO13_GCBOpen/1, DO12_MCBOpen/1
  Constant7/1 -> DO14/2, DO15/2, DO13_GCBOpen/2, DO12_MCBOpen/2
  DO12_MCBOpen/1 -> Bus Creator3/1  "Gen2_MCBOpen"
  DO13_GCBOpen/1 -> Bus Creator3/2  "Gen2_GCBOpen"
  DO14/1 -> Bus Creator3/3  "Gen2_DI11_MCB_Busbar"
  DO15/1 -> Bus Creator3/4  "Gen2_DI12_GCB_Busbar"
  Bus Creator/1 -> [T0]
  Bus Creator1/1 -> [T1]
  Bus Creator3/1 -> [T3]
  Bus Creator2/1 -> [T2]
  [T0] -> Bus Creator6/1  "00-03"
  [T1] -> Bus Creator6/2  "04-07"
  [T2] -> Bus Creator6/3  "08-11"
  [T3] -> Bus Creator6/4  "12-15"

== system Diesel_UnitTest/SM_DIESEL_UNIT_TEST/Banshee_HWCtrl_IOs/GR1 B AIN (CH00-15) ==
  AnalogIn : rtio_opalrt_common/AnalogIn  CtrlName='OpCtrl'  portNb=1  FcnNos=Slot 1 Module B Subsection 1  size=16  maxcount=8  count=8  numchan=8  sampleTime=0
      settings: AttributesFormatString=%<CtrlName>
  AnalogIn1 : rtio_opalrt_common/AnalogIn  CtrlName='OpCtrl'  portNb=2  FcnNos=Slot 1 Module B Subsection 2  size=16  maxcount=8  count=8  numchan=8  sampleTime=0
      settings: AttributesFormatString=%<CtrlName>
  Mux6 : Mux  Inputs=2
  Terminator2 : Terminator
  Terminator3 : Terminator
  Out1 : Outport
  wires:
  Mux6/1 -> Out1/1
  AnalogIn1/2 -> Terminator3/1
  AnalogIn/2 -> Terminator2/1
  AnalogIn1/1 -> Mux6/2
  AnalogIn/1 -> Mux6/1

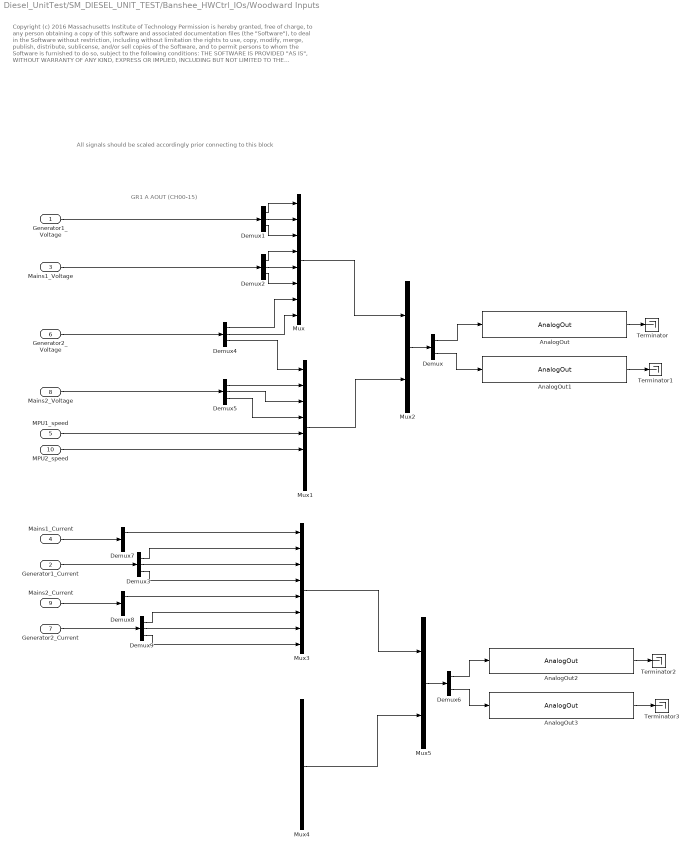
== system Diesel_UnitTest/SM_DIESEL_UNIT_TEST/Banshee_HWCtrl_IOs/Woodward Inputs ==
  note: Copyright (c) 2016 Massachusetts Institute of Technology
      | Permission is hereby granted, free of charge, to any person obtaining a copy of this software and associated documentation files (the "Software"), to deal
      | in the Software without restriction, including without limitation the rights to use, copy, modify, merge, publish, distribute, sublicense, and/or sell copies of the
      | Software, and to permit persons to whom the Software is furnished to do so, subject to the following conditions:
      |
      | THE SOFTWARE IS PROVIDED "AS IS", WITHOUT WARRANTY OF ANY KIND, EXPRESS OR IMPLIED, INCLUDING BUT NOT LIMITED TO THE
      | WARRANTIES OF MERCHANTABILITY, FITNESS FOR A PARTICULAR PURPOSE AND NONINFRINGEMENT. IN NO EVENT SHALL THE AUTHORS
      | OR COPYRIGHT HOLDERS BE LIABLE FOR ANY CLAIM, DAMAGES OR OTHER LIABILITY, WHETHER IN AN ACTION OF CONTRACT, TORT OR
      | OTHERWISE, ARISING FROM, OUT OF OR IN CONNECTION WITH THE SOFTWARE OR THE USE OR OTHER DEALINGS IN THE SOFTWARE
  note: GR1 A AOUT (CH00-15)
  note: All signals should be scaled accordingly prior connecting to this block
  Generator1_Voltage : Inport
  Generator1_Current : Inport  Port=2
  Mains1_Voltage : Inport  Port=3
  Mains1_Current : Inport  Port=4
  MPU1_speed : Inport  Port=5
  Generator2_Voltage : Inport  Port=6
  Generator2_Current : Inport  Port=7
  Mains2_Voltage : Inport  Port=8
  Mains2_Current : Inport  Port=9
  MPU2_speed : Inport  Port=10
  AnalogOut : rtio_opalrt_common/AnalogOut  CtrlName='OpCtrl'  portNb=1  FcnNos=Slot 1 Module A Subsection 1  size=16  maxcount=8  count=8  numchan=8  israngeinput=off  voltagerange=[-16 ... 16]  slot=0  side=0  mismatch=0  slotside=Slot_1_Module_A
      settings: AttributesFormatString=%<CtrlName>
  AnalogOut1 : rtio_opalrt_common/AnalogOut  CtrlName='OpCtrl'  portNb=2  FcnNos=Slot 1 Module A Subsection 2  size=16  maxcount=8  count=8  numchan=8  israngeinput=off  voltagerange=[-16 ... 16]  slot=0  side=0  mismatch=0  slotside=Slot_1_Module_A
      settings: AttributesFormatString=%<CtrlName>
  AnalogOut2 : rtio_opalrt_common/AnalogOut  CtrlName='OpCtrl'  portNb=3  FcnNos=Slot 2 Module A Subsection 1  size=16  maxcount=8  count=8  numchan=8  israngeinput=off  voltagerange=[-16 ... 16]  slot=1  side=0  mismatch=0  slotside=Slot_2_Module_A
      settings: AttributesFormatString=%<CtrlName>
  AnalogOut3 : rtio_opalrt_common/AnalogOut  CtrlName='OpCtrl'  portNb=4  FcnNos=Slot 2 Module A Subsection 2  size=16  maxcount=8  count=8  numchan=8  israngeinput=off  voltagerange=[-16 ... 16]  slot=1  side=0  mismatch=0  slotside=Slot_2_Module_A
      settings: AttributesFormatString=%<CtrlName>
  Demux : Demux  Outputs=2
  Demux{1..5,7..9} (8 alike) : Demux  Outputs=3
  Demux6 : Demux  Outputs=2
  Mux{,1,3..4} (4 alike) : Mux  Inputs=8
  Mux2 : Mux  Inputs=2
  Mux5 : Mux  Inputs=2
  Terminator{,1..3} (4 alike) : Terminator
  wires:
  Mains1_Voltage/1 -> Demux2/1
  Generator1_Voltage/1 -> Demux1/1
  Mux2/1 -> Demux/1
  Mux1/1 -> Mux2/2
  Mux/1 -> Mux2/1
  Demux/2 -> AnalogOut1/1
  Demux/1 -> AnalogOut/1
  AnalogOut1/1 -> Terminator1/1
  AnalogOut/1 -> Terminator/1
  Demux1/1 -> Mux/1
  Demux1/2 -> Mux/2
  Demux1/3 -> Mux/3
  Demux2/1 -> Mux/4
  Demux2/2 -> Mux/5
  Demux2/3 -> Mux/6
  MPU1_speed/1 -> Mux1/5
  Demux4/1 -> Mux/7
  Demux4/2 -> Mux/8
  Demux4/3 -> Mux1/1
  Demux5/1 -> Mux1/2
  Demux5/2 -> Mux1/3
  Demux5/3 -> Mux1/4
  Mux5/1 -> Demux6/1
  Mux4/1 -> Mux5/2
  Mux3/1 -> Mux5/1
  Demux6/2 -> AnalogOut3/1
  Demux6/1 -> AnalogOut2/1
  AnalogOut3/1 -> Terminator3/1
  AnalogOut2/1 -> Terminator2/1
  Generator1_Current/1 -> Demux3/1
  Demux3/1 -> Mux3/2
  Demux3/2 -> Mux3/3
  Demux3/3 -> Mux3/4
  Mains1_Current/1 -> Demux7/1
  Demux7/1 -> Mux3/1
  Mains2_Voltage/1 -> Demux5/1
  Generator2_Voltage/1 -> Demux4/1
  MPU2_speed/1 -> Mux1/6
  Mains2_Current/1 -> Demux8/1
  Demux8/1 -> Mux3/5
  Generator2_Current/1 -> Demux9/1
  Demux9/1 -> Mux3/6
  Demux9/2 -> Mux3/7
  Demux9/3 -> Mux3/8

== system Diesel_UnitTest/SM_DIESEL_UNIT_TEST/Banshee_HWCtrl_IOs/Woodward Outputs - Diesel - Gen2 ==
  note: Copyright (c) 2016 Massachusetts Institute of Technology
      | Permission is hereby granted, free of charge, to any person obtaining a copy of this software and associated documentation files (the "Software"), to deal
      | in the Software without restriction, including without limitation the rights to use, copy, modify, merge, publish, distribute, sublicense, and/or sell copies of the
      | Software, and to permit persons to whom the Software is furnished to do so, subject to the following conditions:
      |
      | THE SOFTWARE IS PROVIDED "AS IS", WITHOUT WARRANTY OF ANY KIND, EXPRESS OR IMPLIED, INCLUDING BUT NOT LIMITED TO THE
      | WARRANTIES OF MERCHANTABILITY, FITNESS FOR A PARTICULAR PURPOSE AND NONINFRINGEMENT. IN NO EVENT SHALL THE AUTHORS
      | OR COPYRIGHT HOLDERS BE LIABLE FOR ANY CLAIM, DAMAGES OR OTHER LIABILITY, WHETHER IN AN ACTION OF CONTRACT, TORT OR
      | OTHERWISE, ARISING FROM, OUT OF OR IN CONNECTION WITH THE SOFTWARE OR THE USE OR OTHER DEALINGS IN THE SOFTWARE
  Gen2 MCB Status : Inport
  WoodwardBias : Inport  Port=2
  Bus Creator1 : BusCreator  Inputs=1
  DIO - Gr3 : Subsystem
  DIO - Woodward : Subsystem
  DOUT type config : Subsystem
  Woodward Primary Inputs - Gen2 : Subsystem
  Digital Inputs : Outport
  Gen2 Gov and AVR : Outport  Port=2
  Gen2 Fuel Enable : Outport  Port=3
  Gen2 GCB : Outport  Port=4
  Gen2 MCB : Outport  Port=5
  wires:
  Bus Creator1/1 -> Digital Inputs/1
  DIO - Woodward/1(DIn1) -> DIO - Gr3/1(Dout)
  DIO - Gr3/1(DIn) -> Bus Creator1/1, DIO - Woodward/1(Din_Wood)  "DIN"
  Woodward Primary Inputs - Gen2/1(Gen2 Gov and AVR) -> Gen2 Gov and AVR/1
  DIO - Woodward/3(Gen2 GCB) -> Gen2 GCB/1
  DIO - Woodward/2(Gen2 Fuel Enable) -> Gen2 Fuel Enable/1
  DIO - Woodward/4(Gen2 MCB) -> Gen2 MCB/1
  Gen2 MCB Status/1 -> DIO - Woodward/2(Gen2 MCB Status)
  WoodwardBias/1 -> Woodward Primary Inputs - Gen2/1(WoodwardBias)

== system Diesel_UnitTest/SM_DIESEL_UNIT_TEST/Number of seconds of recording/Increment ==
  Trigger : TriggerPort  VariantControl=Variant
  Increment : Constant
  Memory : Memory  InheritSampleTime=on
  Sum : Sum  Inputs=|++
  Out1 : Outport
  wires:
  Sum/1 -> Out1/1, Memory/1
  Memory/1 -> Sum/1
  Increment/1 -> Sum/2
